simulink model "aero"  (R2025b)
settings: Solver=VariableStepAuto  StartTime=0.0  StopTime=10.0  RelTol=1e-3
settings Model: Creator=shunyu  LastModifiedBy=shunyu

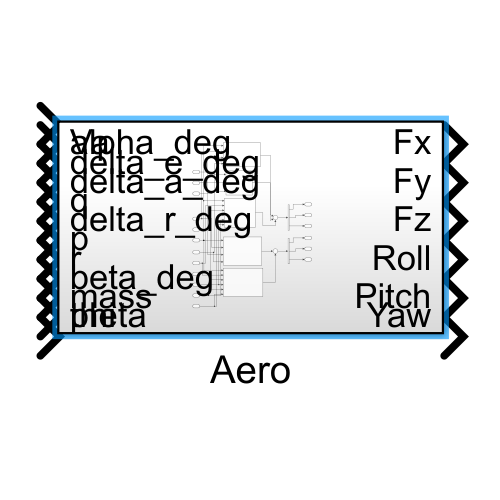
[thumbnail: Simulink's stored preview of the top-level diagram]
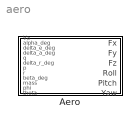
== system aero ==
  Aero : Subsystem

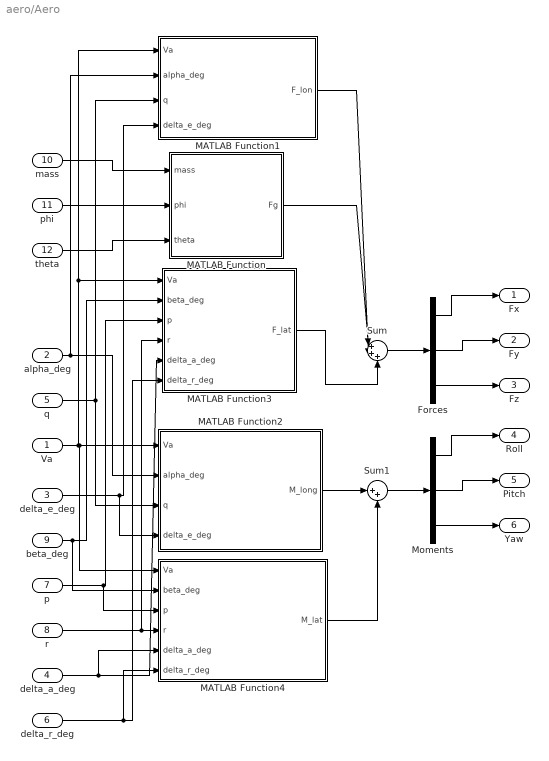
== system aero/Aero ==
  Va : Inport
  alpha_deg : Inport  Port=2
  delta_e_deg : Inport  Port=3
  delta_a_deg : Inport  Port=4
  q : Inport  Port=5
  delta_r_deg : Inport  Port=6
  p : Inport  Port=7
  r : Inport  Port=8
  beta_deg : Inport  Port=9
  mass : Inport  Port=10
  phi : Inport  Port=11
  theta : Inport  Port=12
  Forces : Demux  Outputs=3
  MATLAB Function : MATLAB Function  TreatAsAtomicUnit=on
  MATLAB Function1 : MATLAB Function  TreatAsAtomicUnit=on
  MATLAB Function2 : MATLAB Function  TreatAsAtomicUnit=on
  MATLAB Function3 : MATLAB Function  TreatAsAtomicUnit=on
  MATLAB Function4 : MATLAB Function  TreatAsAtomicUnit=on
  Moments : Demux  Outputs=3
  Sum : Sum  Inputs=|+++
  Sum1 : Sum  Inputs=|++
  Fx : Outport
  Fy : Outport  Port=2
  Fz : Outport  Port=3
  Roll : Outport  Port=4
  Pitch : Outport  Port=5
  Yaw : Outport  Port=6
  wires:
  mass/1 -> MATLAB Function/1(mass)
  delta_r_deg/1 -> MATLAB Function3/6(delta_r_deg), MATLAB Function4/6(delta_r_deg)
  delta_a_deg/1 -> MATLAB Function3/5(delta_a_deg), MATLAB Function4/5(delta_a_deg)
  q/1 -> MATLAB Function1/3(q), MATLAB Function2/3(q)
  delta_e_deg/1 -> MATLAB Function1/4(delta_e_deg), MATLAB Function2/4(delta_e_deg)
  phi/1 -> MATLAB Function/2(phi)
  theta/1 -> MATLAB Function/3(theta)
  Sum1/1 -> Moments/1
  MATLAB Function2/1(M_long) -> Sum1/1
  alpha_deg/1 -> MATLAB Function1/2(alpha_deg), MATLAB Function2/2(alpha_deg)
  Va/1 -> MATLAB Function4/1(Va), MATLAB Function2/1(Va), MATLAB Function1/1(Va), MATLAB Function3/1(Va)
  r/1 -> MATLAB Function4/4(r), MATLAB Function3/4(r)
  p/1 -> MATLAB Function4/3(p), MATLAB Function3/3(p)
  beta_deg/1 -> MATLAB Function3/2(beta_deg), MATLAB Function4/2(beta_deg)
  MATLAB Function1/1(F_lon) -> Sum/2
  MATLAB Function/1(Fg) -> Sum/1
  MATLAB Function3/1(F_lat) -> Sum/3
  MATLAB Function4/1(M_lat) -> Sum1/2
  Sum/1 -> Forces/1
  Forces/1 -> Fx/1
  Forces/2 -> Fy/1
  Forces/3 -> Fz/1
  Moments/1 -> Roll/1
  Moments/2 -> Pitch/1
  Moments/3 -> Yaw/1

== matlab function aero/Aero/MATLAB Function1 ==
  data: Va input; F_lon output; alpha_deg input; q input; delta_e_deg input
function F_lon = computeLongitudinalForces(Va, alpha_deg, q, delta_e_deg)
    alpha = deg2rad(alpha_deg);
    delta_e = deg2rad(delta_e_deg);

    S = GeoConsts.S;
    c = GeoConsts.c;
    AR = GeoConsts.AR;

    Q = 0.5 * 1.225 * Va^2;

    % Stall model
    M = 50;
    alpha0 = 0.47;
    CL_alpha = (pi * AR) / (1 + sqrt(1 + (AR/2)^2));
    sig = (1 + exp(-M*(alpha - alpha0)) + exp(M*(alpha + alpha0))) / ...
          ((1 + exp(-M*(alpha - alpha0))) * (1 + exp(M*(alpha + alpha0))));
    CL_lin = LongitudinalCoeffs.CL0 + CL_alpha * alpha;
    CL_nl  = 2 * sin(alpha) * sin(alpha)^2 * cos(alpha);
    CL = (1 - sig) * CL_lin + sig * CL_nl + ...
         LongitudinalCoeffs.CL_q * (c/(2*Va)) * q + ...
         LongitudinalCoeffs.CL_de * delta_e;

    CD_ind = (CL_lin^2) / (pi * 0.9 * AR);  % e_os = 0.9
    CD = LongitudinalCoeffs.CDp + CD_ind + ...
         LongitudinalCoeffs.CD_q * (c/(2*Va)) * q + ...
         LongitudinalCoeffs.CD_de * abs(delta_e);

    F_lift = Q * S * CL;
    F_drag = Q * S * CD;

    % Convert to body frame
    Fx = -F_drag * cos(alpha) + (-F_lift) * sin(alpha);
    Fz = -F_drag * sin(alpha) - F_lift * cos(alpha);

    F_lon = [Fx; 0; Fz];
end

== matlab function aero/Aero/MATLAB Function ==
  data: mass input; Fg output; phi input; theta input
function Fg = ComputeGravityForce(mass, phi, theta)
g = 9.81;
% Body-frame gravity force components
Fg = mass * g * [-sin(theta);
                 cos(theta)*sin(phi);
                 cos(theta)*cos(phi)];
end

== matlab function aero/Aero/MATLAB Function3 ==
  data: Va input; F_lat output; beta_deg input; p input; r input; delta_a_deg input; delta_r_deg input
function F_lat = computeLateralForces(Va, beta_deg, p, r, delta_a_deg, delta_r_deg)
    beta = deg2rad(beta_deg);
    delta_a = deg2rad(delta_a_deg);
    delta_r = deg2rad(delta_r_deg);

    S = GeoConsts.S;
    b = GeoConsts.b;
    Q = 0.5 * 1.225 * Va^2;

    CY = LateralCoeffs.CY0 + ...
         LateralCoeffs.CY_beta * beta + ...
         LateralCoeffs.CY_p * (b/(2*Va)) * p + ...
         LateralCoeffs.CY_r * (b/(2*Va)) * r + ...
         LateralCoeffs.CY_da * delta_a + ...
         LateralCoeffs.CY_dr * delta_r;

    Fy = Q * S * CY;
    F_lat = [0; Fy; 0];
end

== matlab function aero/Aero/MATLAB Function2 ==
  data: Va input; M_long output; alpha_deg input; q input; delta_e_deg input
function M_long = computeLongitudinalMoment(Va, alpha_deg, q, delta_e_deg)

    alpha = deg2rad(alpha_deg);
    delta_e = deg2rad(delta_e_deg);

    if Va < 1e-3
        Va = 1e-3;
    end

    S = GeoConsts.S;
    c = GeoConsts.c;
    rho = 1.225;

    Q = 0.5 * rho * Va^2;

    Cm = LongitudinalCoeffs.Cm0 + ...
         LongitudinalCoeffs.Cm_alpha * alpha + ...
         LongitudinalCoeffs.Cm_q * (c/(2*Va)) * q + ...
         LongitudinalCoeffs.Cm_de * delta_e;

    My = Q * S * c * Cm;

    M_long = [0; My; 0];
end

== matlab function aero/Aero/MATLAB Function4 ==
  data: Va input; M_lat output; beta_deg input; p input; r input; delta_a_deg input; delta_r_deg input
function M_lat = computeLateralMoments(Va, beta_deg, p, r, delta_a_deg, delta_r_deg)

    beta = deg2rad(beta_deg);
    delta_a = deg2rad(delta_a_deg);
    delta_r = deg2rad(delta_r_deg);

    if Va < 1e-3
        Va = 1e-3;
    end

    S = GeoConsts.S;
    b = GeoConsts.b;
    rho = 1.225;

    Q = 0.5 * rho * Va^2;

    Cl = LateralCoeffs.Cl0 + ...
         LateralCoeffs.Cl_beta * beta + ...
         LateralCoeffs.Cl_p * (b/(2*Va)) * p + ...
         LateralCoeffs.Cl_r * (b/(2*Va)) * r + ...
         LateralCoeffs.Cl_da * delta_a + ...
         LateralCoeffs.Cl_dr * delta_r;

    Cn = LateralCoeffs.Cn0 + ...
         LateralCoeffs.Cn_beta * beta + ...
         LateralCoeffs.Cn_p * (b/(2*Va)) * p + ...
         LateralCoeffs.Cn_r * (b/(2*Va)) * r + ...
         LateralCoeffs.Cn_da * delta_a + ...
         LateralCoeffs.Cn_dr * delta_r;

    Mx = Q * S * b * Cl;
    Mz = Q * S * b * Cn;

    M_lat = [Mx;
             0;
             Mz];
end
